simulink model "AEB_MPC"  (R2021b)
settings: Solver=ode4  StartTime=0.0  StopTime=20  FixedStep=simtime  RelTol=1e-3
InitFcn:
  | clear all
  | 
  | % These are the starting values
  | initial_stopping_distance = 350; % set the stopping distance in m (6.368 and 11 is max deccel -9.5)
  | initial_velocity = 37.77; % set the initial velocity in m/s
  | road_grade = 0; %set road grade in degrees
  | sampletime = 0.01; %set the sample time of the controller
  | Ts = sampletime;
  | simtime = sampletime; %simulation set
  | 
  | initialdeccelcalc = -(initial_velocity^2)/(2*initial_stopping_distance);
libraries: simulink x2, sim3dlib x2, vdynlib x2, sim3dprobsensorlib x1, dspvision x1, autolibshared x1
settings Model: Creator=Tanmay Panchal  LastModifiedBy=Vishal kain
settings SolverCC: AlgebraicLoopSolver=TrustRegion
settings DebuggingCC: SFMachineParentedDataDiag=warning

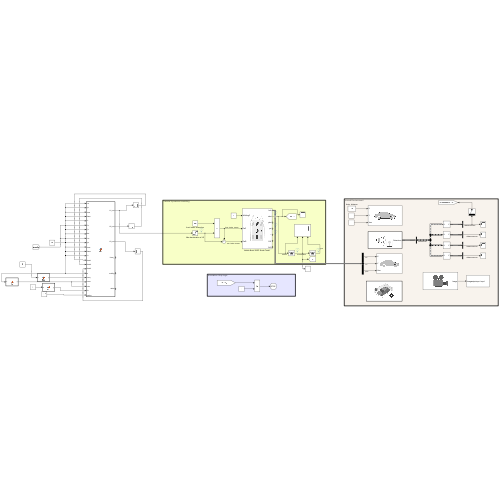
[thumbnail: Simulink's stored preview of the top-level diagram]
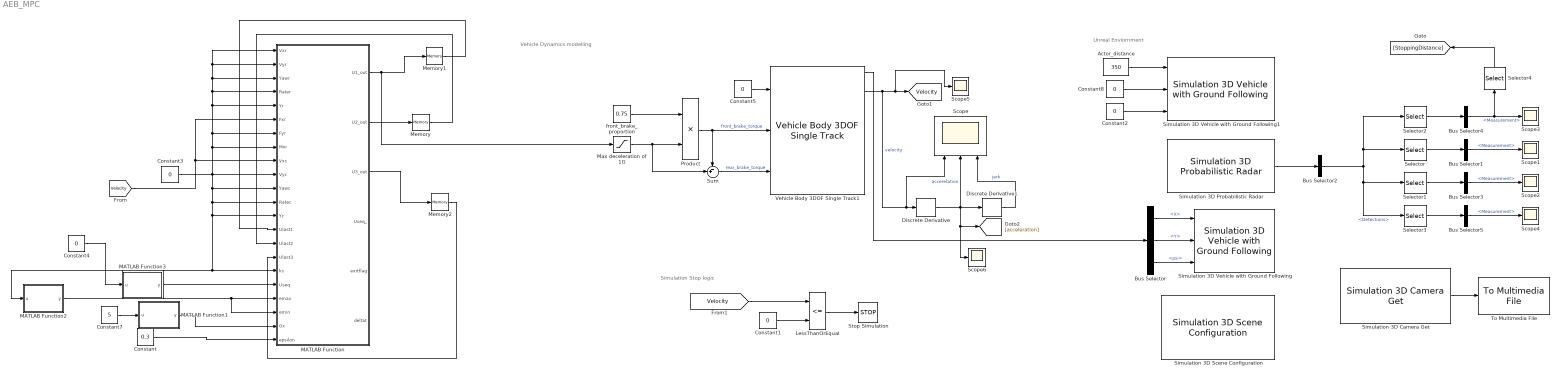
== system AEB_MPC ==
  note: Vehicle Dynamics modelling
  note: Unreal Enviornment
  note: Simulation Stop logic
  Actor_distance : Constant  Value=350
  Bus Selector : BusSelector  OutputSignals=InertFrm.Cg.Disp.X,InertFrm.Cg.Disp.Y,InertFrm.Cg.Ang.psi
  Bus Selector{1,3..5} (4 alike) : BusSelector  OutputSignals=Measurement
  Bus Selector2 : BusSelector  OutputSignals=Detections
  Constant : Constant  Value=0.3
  Constant{1..5,8} (6 alike) : Constant  Value=0
  Constant7 : Constant  Value=5  SampleTime=-1
  Discrete Derivative : simulink/Discrete/Discrete Derivative  gainval=1.0  ICPrevScaledInput=initial_velocity/sampletime  OutMin=[]  OutMax=[]  OutDataType=fixdt(1, 16)  OutScaling=2^-10  DoSatur=off
  Discrete Derivative1 : simulink/Discrete/Discrete Derivative  gainval=1.0  ICPrevScaledInput=0.0  OutMin=[]  OutMax=[]  OutDataType=fixdt(1, 16)  OutScaling=2^-10  DoSatur=off
  LessThanOrEqual : RelationalOperator  Operator=<=  OutDataTypeStr=boolean  RndMeth=Simplest
  MATLAB Function : MATLAB Function  TreatAsAtomicUnit=on
  MATLAB Function1 : MATLAB Function  TreatAsAtomicUnit=on
  MATLAB Function2 : MATLAB Function  TreatAsAtomicUnit=on
  MATLAB Function3 : MATLAB Function  TreatAsAtomicUnit=on
  Max deceleration of 1G : Saturate  UpperLimit=0  LowerLimit=-1605*10
  Memory : Memory
  Memory1 : Memory
  Memory2 : Memory
  Product : Product
  Scope : Scope  NumInputPorts=3
  Scope{1..6} (6 alike) : Scope
  Selector : Selector  InputPortWidth=10  IndexOptions=Index vector (dialog)  Indices=[3]  OutputSizes=1
  Selector1 : Selector  InputPortWidth=10  IndexOptions=Index vector (dialog)  Indices=[5]  OutputSizes=1
  Selector2 : Selector  InputPortWidth=10  IndexOptions=Index vector (dialog)  Indices=[1]  OutputSizes=1
  Selector3 : Selector  InputPortWidth=10  IndexOptions=Index vector (dialog)  Indices=[7]  OutputSizes=1
  Selector4 : Selector  InputPortWidth=3  IndexOptions=Index vector (dialog)  Indices=[1]  OutputSizes=1
  Simulation 3D Camera Get : sim3dlib/Simulation 3D Camera Get  Priority=1  sensorTag=Sim3dSensor3  sensorId=3  sensorName=Sim3dSensor3  vehTagList={'EGOVehicle';'Scene Origin';'Stray'}  vehTag=EGOVehicle  mountLoc=Rearview mirror  offsetFlag=off  tmountOffset=[0, 0, 0]  rmountOffset=[0, 0, 0]  HorizontalResolution=1280  VerticalResolution=720  HorizontalFOV=60  SampleTime=-1  mountPoint=[0.389999985694885 0 1.53999996185303]  mountOrientation=[0 0 0]  aMode=2  ID=3
      settings: SourceProductBaseCode=AE,DR,UV,VE
  Simulation 3D Probabilistic Radar : sim3dprobsensorlib/Simulation 3D Probabilistic Radar  Priority=1  sensorTag=Sim3dSensor1  sensorId=1  sensorName=Sim3dSensor1  vehTagList={'EGOVehicle';'Scene Origin';'Stray'}  vehTag=EGOVehicle  mountLoc=Origin  offsetFlag=off  tmountOffset=[0, 0, 0]  rmountOffset=[0, 0, 0]  AzimuthResolution=4  ElevationResolution=10  RangeResolution=2.5  RangeRateResolution=0.5  AzimuthBiasFraction=0.1  ElevationBiasFraction=0.1  RangeBiasFraction=0.05  RangeRateBiasFraction=0.05  FieldOfView=[ 20, 5 ]  DetectionRange=[ 1, 300 ]  RangeRateLimits=[ -100, 100 ]  DetectionProbability=0.9  FalseAlarmRate=1e-6  ReferenceRange=1000  ReferenceRCS=0  HasElevation=on  HasRangeRate=off  HasNoise=off  HasFalseAlarms=off  InitialSeedSource=Repeatable  InitialSeed=0  MaxNumDetections=10  DetectionCoordinates=Sensor Cartesian  SpecifyOutputBusName=off  BusName=BusSimulation3DRadarTruthSensor  SampleTime=-1  mountPoint=[0 0 0]  mountOrientation=[0 0 0]  aMode=3  ID=1
      settings: SourceProductBaseCode=AE,DR,UV,VE
  Simulation 3D Scene Configuration : sim3dlib/Simulation 3D Scene Configuration  Priority=0  ProjectFormat_internal=Default Scenes  ProjectFormat=Default Scenes  SceneDesc=Straight road  ProjectName=D:\matlab\toolbox\shared\sim3d_projects\automotive_project\UE4\WindowsNoEditor\VehicleSimulation.exe  ScenePath=/Game/Maps/HwStrght  vehTagList={'EGOVehicle';'Scene Origin';'Stray'}  vehTag=EGOVehicle  OpVisEn=off  Ts=0.01  EnableWindow=on  EnableWeather=off  SunAltitude=40.0  SunAzimuth=90  clouds=10  wind=1  fog=0  rain=0  sensorTag=MainCamera1  sensorId=1  sensorName=MainCamera1  mountLoc=Origin  offsetFlag=off  tmountOffset=[0, 0, 0]  rmountOffset=[0, 0, 0]  HorizontalResolution=1280  VerticalResolution=720  HorizontalFOV=60  mountPoint=[0 0 0]  mountOrientation=[0 0 0]  aMode=3  ID=1
      settings: SourceProductBaseCode=AE,DR,UV,VE
  Simulation 3D Vehicle with Ground Following : vdynlib/Vehicle Scenarios/Sim3D/Sim3D Vehicle/Components/Simulation 3D Vehicle with Ground Following  Priority=-1  PassVehMesh=Sport utility vehicle  PassVehMesh_Internal=Sport utility vehicle  MeshPath=/MathWorksSimulation/Vehicles/Muscle/Meshes/SK_MuscleCar.SK_MuscleCar  TrackWidth=1.9  WheelBase=3  WheelRadius=0.35  VehColor=Silver  VehColor_Internal=Silver  InitialPos=[0, 0, 0]  InitialRot=[0, 0, 0]  ActorName=EGOVehicle  VehLightsControl=off  HeadlightColor=[ 1, 1, 1 ]  HighBeamIntensity=100000  LowBeamIntensity=60000  HighBeamConeAngle=1.22  LowBeamConeAngle=1.22  LeftHeadlightOrientation=[ 0, 0 ]  RightHeadlightOrientation=[ 0, 0 ]  BrakelightIntensity=200  ReverselightIntensity=500  SignallightIntensity=500  SignallightPeriod=1  SignalPulseWidth=50  SampleTime=-1  ActorType=SimulinkVehicle  ID=C  aMode=2  ActorTag=EGOVehicle  CoordinateScheme=SAE
      settings: SourceProductBaseCode=VE
  Simulation 3D Vehicle with Ground Following1 : vdynlib/Vehicle Scenarios/Sim3D/Sim3D Vehicle/Components/Simulation 3D Vehicle with Ground Following  Priority=-1  PassVehMesh=Muscle car  PassVehMesh_Internal=Muscle car  MeshPath=/MathWorksSimulation/Vehicles/Muscle/Meshes/SK_MuscleCar.SK_MuscleCar  TrackWidth=1.9  WheelBase=3  WheelRadius=0.35  VehColor=Yellow  VehColor_Internal=Yellow  InitialPos=[0, 5, 0]  InitialRot=[0, 0, 0]  ActorName=Stray  VehLightsControl=off  HeadlightColor=[ 1, 1, 1 ]  HighBeamIntensity=100000  LowBeamIntensity=60000  HighBeamConeAngle=1.22  LowBeamConeAngle=1.22  LeftHeadlightOrientation=[ 0, 0 ]  RightHeadlightOrientation=[ 0, 0 ]  BrakelightIntensity=200  ReverselightIntensity=500  SignallightIntensity=500  SignallightPeriod=1  SignalPulseWidth=50  SampleTime=-1  ActorType=SimulinkVehicle  ID=C  aMode=2  ActorTag=Stray  CoordinateScheme=SAE
      settings: SourceProductBaseCode=VE
  Stop Simulation : Stop
  Sum : Sum  Inputs=-+|
  To Multimedia File : dspvision/To Multimedia File  outputFilename=C:\Autodrive Controls\outputmpc1.mp4  streamSelection=Video only  videoCompressor=None (uncompressed)  audioCompressor=None (uncompressed)  imagePorts=One multidimensional signal  fileType=MPEG4  audioDatatype=Determine from input data type  fourcc=RGB  videoQuality=75  mj2000CompFactor=10
  Vehicle Body 3DOF Single Track1 : autolibshared/Vehicle Body 3DOF Single Track  trackMode=Single (bicycle)  inputMode=External longitudinal forces  frontSteerMode=on  rearSteerMode=off  windMode=off  muMode=off  extFMode=off  extMMode=off  htchFMode=off  htchMMode=off  extXo=off  extpsio=off  extxdoto=off  extro=off  extYo=off  extTamb=off  extydoto=off  aMode=2  NF=2  NR=2  m=1625  a=1.135  b=1.465  h=0.509  dh=1  hh=0.2  X_o=0  xdot_o=initial_velocity  CalphaMode=off  sigmaMode=on  d=0  hl=0  w=[1.4,1.4]  Cy_f=12e3  Cy_r=11e3  sigma_f=.1  sigma_r=.1  alpha_f_brk=[-.1 .1]  Cy_f_data=[-9e3 9e3]  alpha_r_brk=[-.1 .1]  Cy_r_data=[-9e3 9e3]  Y_o=0  ydot_o=0  Izz=2045  psi_o=0  r_o=0  Af=2  Cd=.3  Cl=.1  Cpm=.1  beta_w=[0:0.01:0.3]  Cs=[0:0.03:0.9]  Cym=[0:0.01:0.3]  Pabs=101325  Tair=273  g=9.81  mu=1  xdot_tol=.01  Fznom=5000  Fxtire_sat=7e4  Fytire_sat=7e4  longOff=0  latOff=0  vertOff=0  wrapAng=off
      settings: SourceProductBaseCode=PW,DR,MT,UV,VE
  front_brake_proportion : Constant  Value=0.75
  tag scope: Velocity=global
  wires:
  Discrete Derivative/1 -> Scope6/1, [acceleration], Discrete Derivative1/1, Scope/2  "accerelation"
  Vehicle Body 3DOF Single Track1/2 -> Scope/1, Discrete Derivative/1, Scope5/1, [Velocity]  "velocity"
  Discrete Derivative1/1 -> Scope/3  "jerk"
  LessThanOrEqual/1 -> Stop Simulation/1
  [Velocity] -> LessThanOrEqual/1
  Constant5/1 -> Vehicle Body 3DOF Single Track1/1
  MATLAB Function/1(U1_out) -> Memory1/1, Max deceleration of 1G/1
  Max deceleration of 1G/1 -> Sum/2, Product/2
  Sum/1 -> Vehicle Body 3DOF Single Track1/3  "rear_brake_torque"
  front_brake_proportion/1 -> Product/1
  Product/1 -> Sum/1, Vehicle Body 3DOF Single Track1/2  "front_brake_torque"
  Bus Selector/2 -> Simulation 3D Vehicle with Ground Following/2  "<Y>"
  Bus Selector/1 -> Simulation 3D Vehicle with Ground Following/1  "<X>"
  Bus Selector/3 -> Simulation 3D Vehicle with Ground Following/3  "<psi>"
  Constant2/1 -> Simulation 3D Vehicle with Ground Following1/3
  Constant8/1 -> Simulation 3D Vehicle with Ground Following1/2
  Actor_distance/1 -> Simulation 3D Vehicle with Ground Following1/1
  Simulation 3D Probabilistic Radar/1 -> Bus Selector2/1
  Bus Selector2/1 -> Selector/1, Selector2/1, Selector3/1, Selector1/1  "<Detections>"
  Selector/1 -> Bus Selector1/1
  Bus Selector1/1 -> Scope1/1  "<Measurement>"
  Bus Selector3/1 -> Scope2/1  "<Measurement>"
  Selector1/1 -> Bus Selector3/1
  Selector2/1 -> Bus Selector4/1
  Bus Selector4/1 -> Scope3/1, Selector4/1  "<Measurement>"
  Bus Selector5/1 -> Scope4/1  "<Measurement>"
  Selector3/1 -> Bus Selector5/1
  Selector4/1 -> [StoppingDistance]
  Simulation 3D Camera Get/1 -> To Multimedia File/1
  Constant1/1 -> LessThanOrEqual/2
  Constant/1 -> MATLAB Function/22(epsilon)
  Constant3/1 -> MATLAB Function/8(Mxr), MATLAB Function/7(Fyr), MATLAB Function/5(Yr), MATLAB Function/4(Rater), MATLAB Function/3(Yawr), MATLAB Function/1(Vxr), MATLAB Function/2(Vyr), MATLAB Function/17(ks), MATLAB Function2/1(u), MATLAB Function/13(Yc), MATLAB Function/12(Ratec), MATLAB Function/11(Yawc), MATLAB Function/10(Vyc)
  Constant7/1 -> MATLAB Function1/1(u)
  MATLAB Function1/1(y) -> MATLAB Function/21(Gx)
  [Velocity] -> MATLAB Function/6(Fxr), MATLAB Function/9(Vxc)
  MATLAB Function2/1(y) -> MATLAB Function/19(emax), MATLAB Function/20(emin)
  Memory1/1 -> MATLAB Function/14(Ulast1)
  MATLAB Function/2(U2_out) -> Memory/1
  Memory/1 -> MATLAB Function/15(Ulast2)
  MATLAB Function/3(U3_out) -> Memory2/1
  Memory2/1 -> MATLAB Function/16(Ulast3)
  MATLAB Function3/1(y) -> MATLAB Function/18(Useq)
  Constant4/1 -> MATLAB Function3/1(u)
  Vehicle Body 3DOF Single Track1/1 -> Bus Selector/1

== matlab function AEB_MPC/MATLAB Function1 ==
  data: u input; y output
function y = fcn(u)

y = u*ones(70,1);

== matlab function AEB_MPC/MATLAB Function ==
  data: Vxr input; U1_out output; Vyr input; Yawr input; Rater input; Yr input; Fxr input; Fyr input; Mxr input; Vxc input; Vyc input; Yawc input; Ratec input; Yc input; Ulast1 input; Ulast2 input; Ulast3 input; ks input; Useq input; emax input; emin input; Gx input; epsilon input; U2_out output; U3_out output; Useq_ output; exitflag output; deltat output
function [U1_out, U2_out, U3_out, Useq_, exitflag, deltat] = ...
    mPc(Vxr,Vyr,Yawr,Rater,Yr,Fxr,Fyr,Mxr,Vxc,Vyc,Yawc,Ratec,Yc,...
    Ulast1,Ulast2,Ulast3,ks,Useq,emax,emin,Gx,epsilon) %#ok<STOUT> 
%Vyr lateral velocity, Yawr yaw angle, Rater yaw rate, Yr lateral position
%Fyr lateral force in front tyre,Mxr moment generated by longitudinal force
%'r'means reference | | 'c'means current

    tstart=tic;%timing on
    if Vxc<0.2
        Vxc=0.2;%make sure many expressions' denominator isn't 0 11 end
    end
    lr=1.67;
    threshold=0.1022;
    miu=0.7;
    rmax=9.81*miu/Vxc;
    %% Initilization
    Nx=5;%number of state
    Nu=3;%number of control
    Np=70;%prediction horizon
    %N1 cannot be equal to N2
    Nc=6;%control horizon
    N1=40;
    N2=10;
    % N3=20;
    %reference
    r=zeros(Nx,1);%state reference
    r(1)=Vxr;
    r(2)=Vyr;
    r(3)=Yawr;
    r(4)=Rater;
    r(5)=Yr;
    ur1=Fxr;
    ur2=Fyr;
    ur3=Mxr;%control reference

    %states
    x=zeros(Nx,1);%state reference
    x(1)=Vxc;
    x(2)=Vyc;
    x(3)=Yawc;
    x(4)=Ratec;
    x(5)=Yc;

    %control
    u=zeros(Nu,1);%state reference
    u(1)=Ulast1;
    u(2)=Ulast2;
    u(3)=Ulast3;

    %get augmented states
    kesi=zeros(Nx+Nu,1);%[X;U]
    kesi(1)=x(1)-r(1);
    kesi(2)=x(2)-r(2);
    kesi(3)=x(3)-r(3);
    kesi(4)=x(4)-r(4);
    kesi(5)=x(5)-r(5);
    kesi(6)=u(1)-ur1;
    kesi(7)=u(2)-ur2;
    kesi(8)=u(3)-ur3;

    Ts1=0.05;%sample time
    Ts2=0.2;

    %% Modellng->Discretization->prediction->quadratic programming
    %Modelling&Linearization&Discretization
    steps=Np+1;
    A = zeros(Nx+Nu,Nx+Nu,steps);
    B = zeros(Nx+Nu,Nu*2,steps);
    Dc = zeros(Nx+Nu,1,steps);
    C=[1 0 0 0 0 0 0 0;0 1 0 0 0 0 0 0;0 0 1 0 0 0 0 0;0 0 0 1 0 0 0 ...
        0;0 0 0 0 1 0 0 0];

    for ct = 1:steps
        uk = Useq(ct,:);
        if ct == steps
            uk1 = Useq(ct,:);
        else
            uk1= Useq(ct+1,:);
        end
        uk=uk';
        uk1=uk1';
        if ct<N1 %in short prediction region, using zero order hold
            Ts=Ts1;
            m = 1625; %mass
            Iz = 2045; %rotational inertia
            lf = 1.135; % distance from front axle to the mass center
            lr = 1.465; % distance from rear axle to the mass center
            C_a = 12e3; % rear cornering stiffness

            %Enviroment parameters
            miu = 0.7; %frction cooeficient 0.7 for dry road and 0.4 for wet
            g = 9.81; % gravity
            Fz = m*g*lf/(lf+lr); % the load that beared by the rear tire
            %calculate alpha
            Vx = x(1); %longitudinal velocity
            Vy = x(2); %lateral velocity
            r = x(3); %yaw rate
            alphar = Vy/Vx-lr*r/Vx; %calculate linearzing point
            %tire model
            threshold = atan(3*miu*Fz/C_a); % threshold for the tire linear region
            if abs(alphar)<threshold
                %the rear lateral force value (f(x0)) at the linearzing point
                Fyr = -C_a*tan(alphar )+C_a^2/(3*miu*Fz)*abs(tan(alphar ))*tan(alphar ) - ...
                    C_a^3/(27*miu^2*Fz^2)*tan(alphar)^3;
                %the slope of linearized model (f'(x0))
                if alphar>0
                    Cr = -C_a*sec(alphar )^2+C_a^2/(3*miu*Fz)*(2*sec(alphar)^2*tan(alphar)) - ...
                        C_a^3/(27*miu^2*Fz^2)*(3*tan(alphar)^2*sec(alphar)^2);
                else
                    Cr = -C_a*sec(alphar)^2-C_a^2/(3*miu*Fz)*(2*sec(alphar)^2*tan(alphar)) - ...
                        C_a^3/(27*miu^2*Fz^2)*(3*tan(alphar)^2*sec(alphar)^2);
                end
            else
                %the saturation region of tire model
                Fyr = -miu*Fz*sign(alphar);
                Cr = 0;
            end
            %Continuous-time model
            Ac = [0 r Vy 0 0; -r+(Cr*(lr*r-Vy)/(m*Vx^2)) Cr/(m*Vx) -lr*Cr /(m*Vx)-Vx 0 0;...
                lr*Cr*(Vy-lr*r)/(Iz*Vx^2) -lr*Cr/(Iz*Vx) lr^2*Cr/(Iz*Vx) 0 0; -ks 0 1 0 0; 0 1 0 Vx 0 ];

            Bc = [1/m 0 0; 0 1/m 0; 0 lf/Iz 1/Iz; 0 0 0; 0 0 0];
            dcc = [0; (Fyr -Cr *alphar )/m; -lr*(Fyr -Cr *alphar )/Iz; -Vx*ks; 0];

            % dcc = dcc-Ac(1:5,1)*Vx;%adjust the Vx's linearization point
            G = [Ac Bc dcc;zeros(4,9)];
            M = expm(G*Ts);
            Ad = M(1:5,1:5);
            Bd = M(1:5,6:8);
            DK = M(1:5,9);
            deltax = Ad*x+Bd*u+DK-x;
            A(:,:,ct)=[Ad,Bd;zeros(Nu,Nx),eye(Nu)];
            B(:,:,ct)=[Bd zeros(Nx,Nu);eye(Nu) zeros(Nu,Nu)];%in order ...
            %to fit the dimension of B from ZOH with B from FOH, ...
            % augumentation is done here
            Dc(:,:,ct)=[DK;zeros(Nu,1)];%constant component
        elseif ct<N1+N2 %in correction prediction region, using first order hold
            Ts=Ts1+(Ts2-Ts1)*(ct-N1)/(N2-N1);%get this step's correction sample time
            m = 1625; %mass
            Iz = 2045; %rotational inertia
            lf = 1.135; % distance from front axle to the mass center
            lr = 1.465; % distance from rear axle to the mass center
            C_a = 12e3; % rear cornering stiffness
            %Enviroment parameters
            miu = 0.7; %frction cooeficient 0.7 for dry road and 0.4 for wet
            g = 9.81; % gravity
            Fz = m*g*lf/(lf+lr); % the load that beared by the rear tire
            %calculate alpha
            Vx = x(1); %longitudinal velocity
            Vy = x(2); %lateral velocity
            r = x(3); %yaw rate
            alphar = Vy/Vx-lr*r/Vx; %calculate linearzing point
            %tire model
            threshold = atan(3*miu*Fz/C_a); % threshold for the tire linear region
            if abs(alphar)<threshold
                %the rear lateral force value (f(x0)) at the linearzing point
                Fyr = -C_a*tan(alphar)+C_a^2/(3*miu*Fz)*abs(tan(alphar))*tan(alphar) ...
                    -C_a^3/(27*miu^2*Fz^2)*tan(alphar)^3;
                %the slope of linearized model (f'(x0))
                if alphar > 0
                    Cr = -C_a*sec(alphar)^2+C_a^2/(3*miu*Fz)*(2*sec(alphar)^2*tan(alphar)) - ...
                        C_a^3/(27*miu^2*Fz^2)*(3*tan(alphar)^2*sec(alphar)^2);
                else
                    Cr = -C_a*sec(alphar)^2 - C_a^2/(3*miu*Fz)*(2*sec(alphar)^2*tan(alphar))...
                        -C_a^3/(27*miu^2*Fz^2)*(3*tan(alphar)^2*sec(alphar)^2);
                end
            else
                %the saturation region of tire model
                Fyr = -miu*Fz*sign(alphar);
                Cr = 0;
            end

            %Continuous-time model
            Ac = [0 r Vy 0 0; -r+(Cr*(lr*r-Vy)/(m*Vx^2)) Cr/(m*Vx) -lr*Cr/(m*Vx)-Vx 0 0 ;...
                lr*Cr*(Vy-lr*r)/(Iz*Vx^2) -lr*Cr/(Iz*Vx) lr^2*Cr/(Iz*Vx) 0 0 ;...
                -ks 0 1 0 0; 0 1 0 Vx 0];
            Bc = [1/m 0 0; 0 1/m 0; 0 lf/Iz 1/Iz; 0 0 0; 0 0 0];
            dcc = [0; (Fyr-Cr*alphar)/m; -lr*(Fyr-Cr*alphar)/Iz; -Vx*ks; 0];
            LAMDA=[Ac Bc dcc zeros(5,4); zeros(4,9) 1/Ts*eye(4); zeros(4,13)];
            M = expm(LAMDA*Ts);
            Ad = M(1:5,1:5);
            PHI1 = M(1:5,6:9);
            PHI2 = M(1:5,10:13);
            Bd1 = (PHI1-PHI2)*[eye(3);zeros(1,3)];
            Bd2 = PHI2*[eye(3);zeros(1,3)];
            DK = PHI1*[0;0;0;1];
            deltax = Ad*x+Bd1*uk+Bd2*uk1+DK-x;
            %%x(k+1)=A*x(k)+B1*u(k)=B2*u(k+1)+DK
            A(:,:,ct)=[Ad Bd1+Bd2;zeros(Nu,Nx) eye(Nu)];
            B(:,:,ct)=[Bd1+Bd2 Bd2;eye(Nu) zeros(Nu,Nu)];
            Dc(:,:,ct)=[DK;zeros(Nu,1)];
        else %in long prediction region, using first order hold
            Ts=Ts2;
            m = 1625; %mass
            Iz = 2045; %rotational inertia
            lf = 1.135; % distance from front axle to the mass center
            lr = 1.465; % distance from rear axle to the mass center
            C_a = 12e3; % rear cornering stiffness

            %Enviroment parameters
            miu = 0.7; %frction cooeficient 0.7 for dry road and 0.4 for wet
            g = 9.81; % gravity
            Fz = m*g*lf/(lf+lr); % the load that beared by the rear tire
            %calculate alpha
            Vx = x(1); %longitudinal velocity
            Vy = x(2); %lateral velocity
            r = x(3); %yaw rate
            alphar = Vy/Vx-lr*r/Vx; %calculate linearzing point
            %tire model
            threshold = atan(3*miu*Fz/C_a); % threshold for the tire linear region
            if abs(alphar)<threshold
                %the rear lateral force value (f(x0)) at the linearzing point
                Fyr = -C_a*tan(alphar)+C_a^2/(3*miu*Fz)*abs(tan(alphar))*tan(alphar) ...
                    -C_a^3/(27*miu^2*Fz^2)*tan(alphar)^3;
                %the slope of linearized model (f'(x0))
                if alphar > 0
                    Cr = -C_a*sec(alphar)^2+C_a^2/(3*miu*Fz)*(2*sec(alphar)^2*tan(alphar)) - ...
                        C_a^3/(27*miu^2*Fz^2)*(3*tan(alphar)^2*sec(alphar)^2);
                else
                    Cr = -C_a*sec(alphar)^2 - C_a^2/(3*miu*Fz)*(2*sec(alphar)^2*tan(alphar))...
                        -C_a^3/(27*miu^2*Fz^2)*(3*tan(alphar)^2*sec(alphar)^2);
                end
            else
                %the saturation region of tire model
                Fyr = -miu*Fz*sign(alphar);
                Cr = 0;
            end

            %Continuous-time model
            Ac = [0 r Vy 0 0; -r+(Cr*(lr*r-Vy)/(m*Vx^2)) Cr/(m*Vx) -lr*Cr/(m*Vx)-Vx 0 0 ;...
                lr*Cr*(Vy-lr*r)/(Iz*Vx^2) -lr*Cr/(Iz*Vx) lr^2*Cr/(Iz*Vx) 0 0 ;...
                -ks 0 1 0 0; 0 1 0 Vx 0];
            Bc = [1/m 0 0; 0 1/m 0; 0 lf/Iz 1/Iz; 0 0 0; 0 0 0];
            dcc = [0; (Fyr-Cr*alphar)/m; -lr*(Fyr-Cr*alphar)/Iz; -Vx*ks; 0];
            LAMDA=[Ac Bc dcc zeros(5,4); zeros(4,9) 1/Ts*eye(4); zeros(4,13)];
            M = expm(LAMDA*Ts);
            Ad = M(1:5,1:5);
            PHI1 = M(1:5,6:9);
            PHI2 = M(1:5,10:13);
            Bd1 = (PHI1-PHI2)*[eye(3);zeros(1,3)];
            Bd2 = PHI2*[eye(3);zeros(1,3)];
            DK = PHI1*[0;0;0;1];
            deltax = Ad*x+Bd1*uk+Bd2*uk1+DK-x;
            %%x(k+1)=A*x(k)+B1*u(k)=B2*u(k+1)+DK
            A(:,:,ct)=[Ad Bd1+Bd2;zeros(Nu,Nx) eye(Nu)];
            B(:,:,ct)=[Bd1+Bd2 Bd2;eye(Nu) zeros(Nu,Nu)];
            Dc(:,:,ct)=[DK;zeros(Nu,1)];
            A(:,:,ct)=[Ad Bd1+Bd2;zeros(Nu,Nx) eye(Nu)];
            B(:,:,ct)=[Bd1+Bd2 Bd2;eye(Nu) zeros(Nu,Nu)];
            Dc(:,:,ct)=[DK;zeros(Nu,1)];
        end
        x=x+deltax; %predict next step's states
    end

    %construct important matrix
    %Y=PHI*kesi+THETA*∆ U+OMEGA*D
    coder.varsize('PHI',[Np*Nx,Nx+Nu]);
    coder.varsize('THETA',[Np*Nx,Nc*Nu]);
    coder.varsize('D',[Np*(Nx+Nu),1]);
    coder.varsize('DD',[Np*Nx,1]);
    coder.varsize('OMEGA',[Nx*Np,(Nx+Nu)*Np]);
    OMEGA=zeros(Nx*Np,(Nx+Nu)*Np);
    PHI=zeros(Np*Nx,Nx+Nu);
    THETA=zeros(Np*Nx,Nc*Nu);
    D = zeros(Np*(Nx+Nu),1);
    DD = zeros(Np*Nx,1);
    product = eye(Nx+Nu);

    for j=1:Np
        PHI((j-1)*Nx+1:j*Nx,:) = C*A(:,:,j)*product;
        product = A(:,:,j)*product;
        D((j-1)*(Nx+Nu)+1:j*(Nx+Nu),:) = Dc(:,:,j);
    end

    for k=1:Nc/2
        product=eye(Nx+Nu);
        for j=k:Np
            THETA((j-1)*Nx+1:j*Nx,(k-1)*Nu*2+1:k*Nu*2) = C*product*B(:,:,k);
            product = A(:,:,j+1)*product;
        end
    end

    for i=1:Np
        product=eye(Nx+Nu);
        for j=i:Np
            OMEGA((j-1)*Nx+1:j*Nx, (i-1)*(Nx+Nu)+1:i*(Nx+Nu)) = C*product;
            product = A(:,:,j+1)*product;
        end
    end

    DD = OMEGA*D;
    Sigma = tril(ones(Nc,Nc));
    Sigma = kron(Sigma,eye(Nu));
    UT=kron(ones(Nc,1),[u(1);u(2);u(3)]);
    error=PHI*kesi;
    Q=kron(eye(Np),diag([4 0 0 100 4]));
    R=kron(eye(Nc),diag([4e-5 0 4e-5]));
    P=kron(eye(Nc),diag([0 3e-5 8e-5]));
    rou1=3e3;
    rou2=5e4;
    rou3=1e6;
    H = 2*[THETA'*Q*THETA+Sigma'*R*Sigma+P zeros(Nc*Nu,3);zeros(1,Nc*Nu) ...
        rou1 0 0;zeros(1,Nc*Nu) 0 rou2 0;zeros(1,Nc*Nu) 0 0 rou3];
    f=[2*(error'*Q*THETA+(OMEGA*D)'*Q*THETA+UT'*R*Sigma),0,0,0];
    %% constraints
    %inequation
    A_I = tril(ones(Nc,Nc));
    A_I = kron(A_I,eye(Nu));
    Ut=kron(ones(Nc,1),[u(1);u(2);u(3)]);%control in last control step
    umin=[-6816; -1e4; -1e3];
    umax=[6816; 1e4; 1e3];
    Umin=kron(ones(Nc,1),umin);
    Umax=kron(ones(Nc,1),umax);
    coder.varsize('A_cons',[Np*6+Nc*Nu*2+Np,Nc*Nu+3]);
    coder.varsize('b_cons',[Np*6+Nc*Nu*2+Np,1]);

    %add handling envelop constriants & environment envolop &longitudinal
    %position constraints
    gamas=[0 1 -lr 0 0;0 -1 lr 0 0;0 0 1 0 0;0 0 -1 0 0];
    gamae=[0 0 0 0 1;0 0 0 0 -1];
    gamax=[1 0 0 0 0];
    Gs=[Vxc*threshold;Vxc*threshold;rmax;rmax];
    Gamas = kron(eye(Np),gamas);
    Gamae = kron(eye(Np),gamae);
    Gsm = kron(ones(Np,1),Gs);
    A_cons0=[A_I zeros(Nc*Nu,3);-A_I zeros(Nc*Nu,3)];
    b_cons0=[Umax-Ut;-Umin+Ut];
    A_cons1 = [Gamas*THETA -ones(4*Np,1) zeros(4*Np,1) zeros(4*Np,1)];
    b_cons1 = Gsm - Gamas*(PHI*kesi+DD);
    A_cons2 = [Gamae*THETA zeros(2*Np,1) -ones(2*Np,1) zeros(2*Np,1)];
    Gse = zeros(2*Np,1);
    Qw = blkdiag(0.6^2, 0.6^2);
    %x(k+1) = A*x(k)+B*u(k)+D(k)+G*w;
    G = [0.1 0; 0 0; 0 0; 0 0;0 0.1];
    var = zeros(Nx,Nx);
    SIGMA = zeros(Np,1);
    for i = 1:Np
        var = A(1:5,1:5,i)*var*A(1:5,1:5,i)'+G*Qw*G';
        %var is Sigma(k),variance of e(k)
        SIGMA(i,1) = sqrt(var(5,5))';
    end
    nmax = zeros(Np, 1);
    nmin = zeros(Np, 1);
    numcc = 0;
    for i = 1:Np
        if (isnan(emax(i,:))) == 0
            nmax(i,:) = -norminv(1-epsilon, -emax(i,1),SIGMA(i,1));
            %calculate the new bounds with given probability of invalidation
            % disp(['nmax: ', num2str(nmax(j,i))]);
            numcc = numcc+1;
        else
            nmax(i,:) = NaN;
        end
        if (isnan(emin(i,:))) == 0
            nmin(i,:) = norminv(1-epsilon, emin(i,1), SIGMA(i,1));
            %calculate the new bounds with given probability of invalidation
            % disp(['nmin: ', num2str(nmin(j,i))]);
            numcc = numcc+1;
        else
            nmin(i,1) = NaN;
        end
    end
    for i=1:Np
        Gse(2*(i-1)+1,:)=emax(i);
        Gse(2*(i-1)+2,:)=-emin(i);
    end
    b_cons2 = Gse - Gamae*(PHI*kesi+DD);
    A_cons = [A_cons0;A_cons1;A_cons2];
    b_cons = [b_cons0;b_cons1;b_cons2];
    if Vxr==0.1
        Gamax = kron(eye(Np),gamax);
        Gamax = tril(ones(Np,Np))*Gamax;
        A_cons3 = [Ts*Gamax*THETA zeros(Np,1) zeros(Np,1) -ones(Np,1)];
        b_cons3 = Gx-Ts*Gamax*(PHI*kesi+DD);
        A_cons = [A_cons;A_cons3];
        b_cons = [b_cons;b_cons3];
    end

    %upper and lower boundary
    deltaumin=[-1e4; -1e4; -1e3];
    deltaumax=[1e4; 1e4; 1e3];
    M1 = 10;
    M2=10; %slack variable related to enviroment constriants
    M3=10; %slack variable related to longitudinal position constriants
    deltaUmin=kron(ones(Nc,1),deltaumin);
    deltaUmax=kron(ones(Nc,1),deltaumax);
    lb=[deltaUmin;0;0;0];
    ub=[deltaUmax;M1;M2;M3];

    %% solve quadratic programming
    opts = optimoptions('quadprog','Algorithm','active-set');
    x_start = zeros(Nu*Nc+3,1); %+3 corresponds to slack variables
    [X, fval ,exitflag] = quadprog(H,f',A_cons,b_cons,[],[],lb,ub,x_start,opts);

    %% calculate control signal
    U1_out=kesi(6)+X(1)+ur1; %Error plus reference value to get final output value
    U2_out=kesi(7)+X(2)+ur2;
    U3_out=kesi(8)+X(3)+ur3;
    U = [kesi(6)+ur1, kesi(7)+ur2, kesi(8)+ur3];
    Useq_= zeros(Np+1,Nu);
    Xsum = zeros(1,Nu);
    for i=1:Nc
        Xsum = Xsum+[X(3*(i-1)+1) X(3*(i-1)+2) X(3*(i-1)+3)];
        Useq_(i,:)= U + Xsum;
    end
    deltat=toc(tstart);%timing off
end

== matlab function AEB_MPC/MATLAB Function2 ==
  data: u input; y output
function y = fcn(u)

y = u*ones(70,1);;

== matlab function AEB_MPC/MATLAB Function3 ==
  data: u input; y output
function y = fcn(u)

y = u*ones(71,3);
